simulink library "csu_rtk_translational_kinematics_lib"  (R2014b)
settings: Solver=ode45  SolverMode=SingleTasking  StartTime=0.0  StopTime=10.0  RelTol=1e-3
libraries: util_info_lib x2, util_extra_lib x1
settings Model: ExtModeAutoUpdateStatusClock=off  Creator=daniloviazzo  LastModifiedBy=mstewart

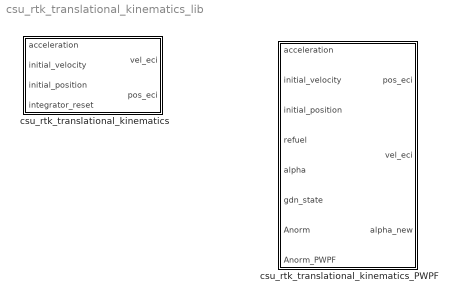
== system csu_rtk_translational_kinematics_lib ==
  csu_rtk_translational_kinematics : Subsystem
  csu_rtk_translational_kinematics_PWPF : Subsystem

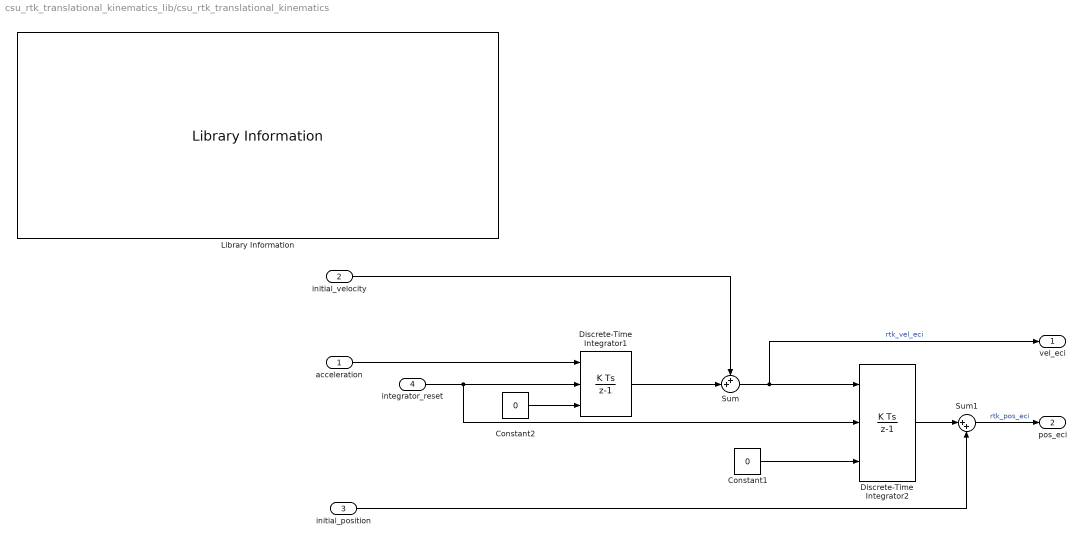
== system csu_rtk_translational_kinematics_lib/csu_rtk_translational_kinematics ==
  acceleration : Inport
  initial_velocity : Inport  Port=2
  initial_position : Inport  Port=3
  integrator_reset : Inport  Port=4
  Constant1 : Constant  Value=0
  Constant2 : Constant  Value=0
  Discrete-Time Integrator1 : DiscreteIntegrator  ExternalReset=rising  InitialConditionSource=external  InitialConditionSetting=Compatibility  SampleTime=-1
  Discrete-Time Integrator2 : DiscreteIntegrator  ExternalReset=rising  InitialConditionSource=external  InitialConditionSetting=Compatibility  SampleTime=-1
  Library Information : util_info_lib/Library Information  owner='NONE'
  Sum : Sum  Inputs=++|
  Sum1 : Sum  Inputs=|++
  vel_eci : Outport
  pos_eci : Outport  Port=2
  wires:
  integrator_reset/1 -> Discrete-Time Integrator1/2, Discrete-Time Integrator2/2
  Discrete-Time Integrator1/1 -> Sum/2
  Discrete-Time Integrator2/1 -> Sum1/1
  initial_velocity/1 -> Sum/1
  Constant2/1 -> Discrete-Time Integrator1/3
  acceleration/1 -> Discrete-Time Integrator1/1
  Sum/1 -> vel_eci/1, Discrete-Time Integrator2/1  "rtk_vel_eci"
  Constant1/1 -> Discrete-Time Integrator2/3
  Sum1/1 -> pos_eci/1  "rtk_pos_eci"
  initial_position/1 -> Sum1/2

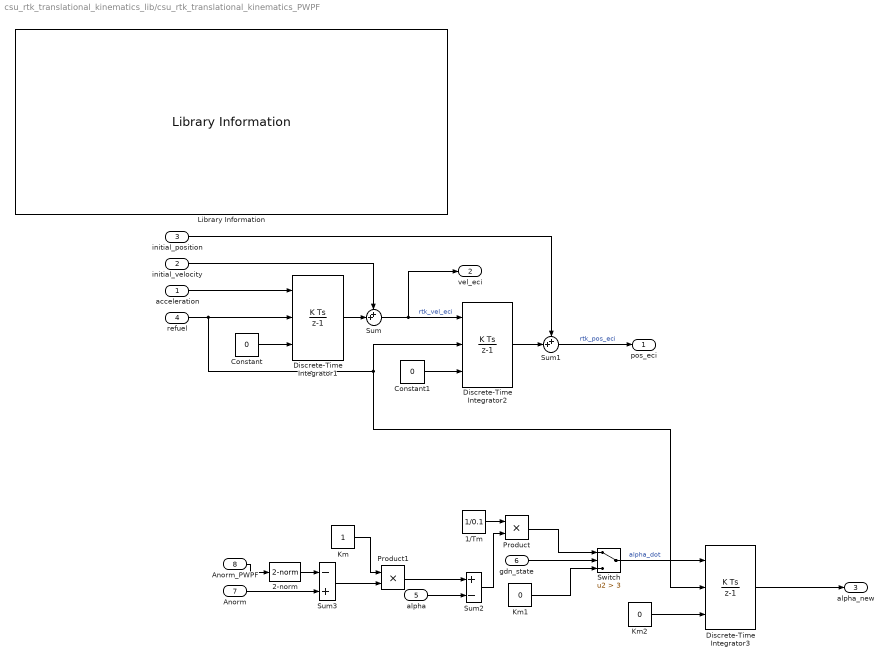
== system csu_rtk_translational_kinematics_lib/csu_rtk_translational_kinematics_PWPF ==
  acceleration : Inport
  initial_velocity : Inport  Port=2
  initial_position : Inport  Port=3
  refuel : Inport  Port=4
  alpha : Inport  Port=5
  gdn_state : Inport  Port=6
  Anorm : Inport  Port=7
  Anorm_PWPF : Inport  Port=8
  1/Tm : Constant  Value=1/0.1
  2-norm : util_extra_lib/2-norm
  Constant : Constant  Value=0
  Constant1 : Constant  Value=0
  Discrete-Time Integrator1 : DiscreteIntegrator  ExternalReset=rising  InitialConditionSource=external  SampleTime=-1
  Discrete-Time Integrator2 : DiscreteIntegrator  ExternalReset=rising  InitialConditionSource=external  SampleTime=-1
  Discrete-Time Integrator3 : DiscreteIntegrator  ExternalReset=rising  InitialConditionSource=external  SampleTime=-1
  Km : Constant
  Km1 : Constant  Value=0
  Km2 : Constant  Value=0
  Library Information : util_info_lib/Library Information  owner='NONE'
  Product : Product  RndMeth=Zero
  Product1 : Product  RndMeth=Zero
  Sum : Sum  Inputs=++|
  Sum1 : Sum  Inputs=++|
  Sum2 : Sum  Inputs=+-
  Sum3 : Sum  Inputs=-+
  Switch : Switch  Criteria=u2 > Threshold  Threshold=3
  pos_eci : Outport
  vel_eci : Outport  Port=2
  alpha_new : Outport  Port=3
  wires:
  Anorm_PWPF/1 -> 2-norm/1
  2-norm/1 -> Sum3/1
  Anorm/1 -> Sum3/2
  Discrete-Time Integrator3/1 -> alpha_new/1
  Km2/1 -> Discrete-Time Integrator3/3
  Switch/1 -> Discrete-Time Integrator3/1  "alpha_dot"
  Product/1 -> Switch/1
  Sum3/1 -> Product1/2
  Product1/1 -> Sum2/1
  Km/1 -> Product1/1
  1/Tm/1 -> Product/1
  Sum2/1 -> Product/2
  alpha/1 -> Sum2/2
  Km1/1 -> Switch/3
  gdn_state/1 -> Switch/2
  Constant/1 -> Discrete-Time Integrator1/3
  refuel/1 -> Discrete-Time Integrator3/2, Discrete-Time Integrator2/2, Discrete-Time Integrator1/2
  acceleration/1 -> Discrete-Time Integrator1/1
  Discrete-Time Integrator1/1 -> Sum/2
  initial_velocity/1 -> Sum/1
  Sum/1 -> Discrete-Time Integrator2/1, vel_eci/1  "rtk_vel_eci"
  Constant1/1 -> Discrete-Time Integrator2/3
  Discrete-Time Integrator2/1 -> Sum1/2
  initial_position/1 -> Sum1/1
  Sum1/1 -> pos_eci/1  "rtk_pos_eci"
